simulink model "Trafo_SIMULINK"  (R2022b)
settings: Solver=FixedStepAuto  StartTime=0.0  StopTime=5  FixedStep=0.00001  RelTol=1e-3
values from neighbouring files (symbols this model uses):
  Ct = 1/(Xt*2*pi*f)    (= 9.94718394324e-05)    [Trafo.m]
  k12 = 120/240    (= 0.5)    [Trafo.m]
  k21 = 240/120    (= 2)    [Trafo.m]
  L12 = 0.149*10^-3    (= 0.000149)    [Trafo.m]
  Lm = 1.88    [Trafo.m]
  Lt = Xt/(2*pi*f)    (= 0.101859163579)    [Trafo.m]
  r1 = 0.25    [Trafo.m]
  r2 = 0.134    [Trafo.m]
  Rt = 32    [Trafo.m]
  Umax = 220    [Trafo.m]
  w = 2*pi*50    (= 314.159265359)    [Trafo.m]
settings Model: Creator=Student  LastModifiedBy=petar
settings SolverCC: AlgebraicLoopSolver=TrustRegion
settings DataIOCC: ReturnWorkspaceOutputs=off
settings DebuggingCC: UnconnectedInputMsg=warning  UnconnectedOutputMsg=warning  UnconnectedLineMsg=warning  SFMachineParentedDataDiag=warning  ArithmeticOperatorsInVariantConditions=warning
settings ModelReferenceCC: EnableRefExpFcnMdlSchedulingChecks=on
settings SFSimCC: CustomCodeUndefinedFunction=UseInterfaceOnly

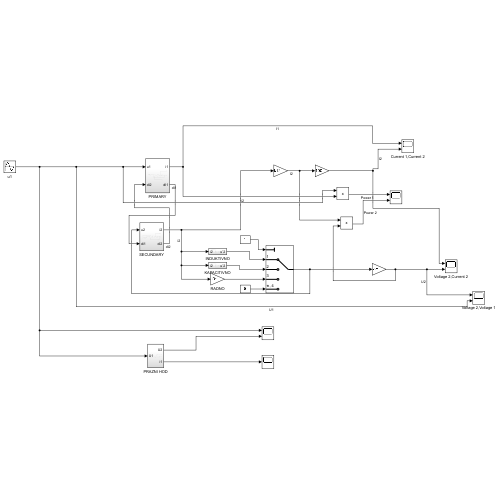
[thumbnail: Simulink's stored preview of the top-level diagram]
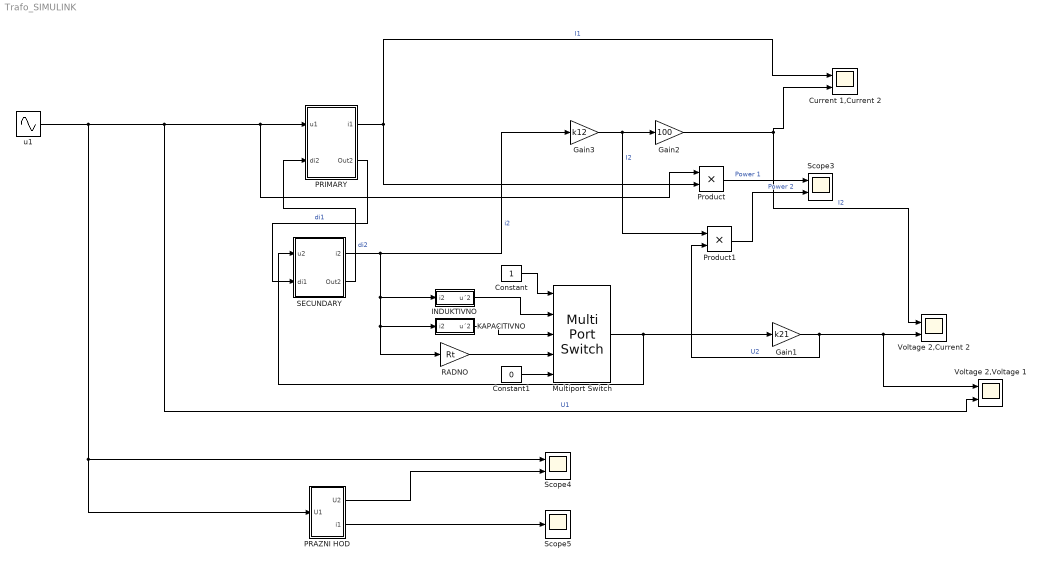
== system Trafo_SIMULINK ==
  Constant : Constant
  Constant1 : Constant  Value=0
  Current 1,Current 2 : Scope  NumInputPorts=2
  Gain1 : Gain  Gain=k21
  Gain2 : Gain  Gain=100
  Gain3 : Gain  Gain=k12
  INDUKTIVNO : Subsystem
  KAPACITIVNO : Subsystem
  Multiport Switch : MultiPortSwitch  Inputs=4  SaturateOnIntegerOverflow=off  InputSameDT=off
  PRAZNI HOD : Subsystem
  PRIMARY : Subsystem
  Product : Product
  Product1 : Product
  RADNO : Gain  Gain=Rt
  SECUNDARY : Subsystem
  Scope3 : Scope  NumInputPorts=2
  Scope4 : Scope  NumInputPorts=2
  Scope5 : Scope
  Voltage 2,Current 2 : Scope  NumInputPorts=2
  Voltage 2,Voltage 1 : Scope  NumInputPorts=2
  u1 : Sin  Amplitude=Umax  Frequency=w  SampleTime=0
  wires:
  u1/1 -> Product/1, PRIMARY/1(u1), Voltage 2,Voltage 1/2, PRAZNI HOD/1(U1), Scope4/1  "U1"
  Gain1/1 -> Product1/2, Voltage 2,Current 2/2, Voltage 2,Voltage 1/1  "U2"
  Gain3/1 -> Product1/1, Gain2/1  "I2"
  PRIMARY/1(i1) -> Current 1,Current 2/1, Product/2  "I1"
  SECUNDARY/1(i2) -> RADNO/1, KAPACITIVNO/1(i2), INDUKTIVNO/1(i2), Gain3/1  "i2"
  PRIMARY/2(Out2) -> SECUNDARY/2(di1)  "di1"
  SECUNDARY/2(Out2) -> PRIMARY/2(di2)  "di2"
  KAPACITIVNO/1(u´2) -> Multiport Switch/3
  INDUKTIVNO/1(u´2) -> Multiport Switch/2
  Multiport Switch/1 -> SECUNDARY/1(u2), Gain1/1
  RADNO/1 -> Multiport Switch/4
  Constant/1 -> Multiport Switch/1
  Gain2/1 -> Current 1,Current 2/2, Voltage 2,Current 2/1  "I2"
  Constant1/1 -> Multiport Switch/5
  Product/1 -> Scope3/1  "Power 1"
  Product1/1 -> Scope3/2  "Power 2"
  PRAZNI HOD/1(U2) -> Scope4/2
  PRAZNI HOD/2(i1) -> Scope5/1

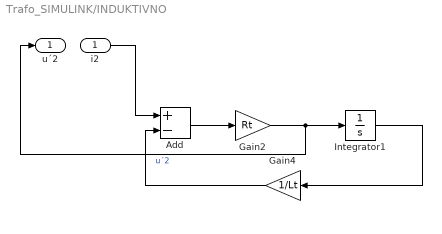
== system Trafo_SIMULINK/INDUKTIVNO ==
  i2 : Inport
  Add : Sum  Inputs=+-
  Gain2 : Gain  Gain=Rt
  Gain4 : Gain  Gain=1/Lt
  Integrator1 : Integrator
  u´2 : Outport  VectorParamsAs1DForOutWhenUnconnected=off
  wires:
  Gain4/1 -> Add/2
  Integrator1/1 -> Gain4/1
  Gain2/1 -> u´2/1, Integrator1/1  "u´2"
  Add/1 -> Gain2/1
  i2/1 -> Add/1

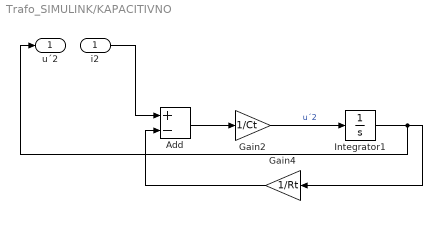
== system Trafo_SIMULINK/KAPACITIVNO ==
  i2 : Inport
  Add : Sum  Inputs=+-
  Gain2 : Gain  Gain=1/Ct
  Gain4 : Gain  Gain=1/Rt
  Integrator1 : Integrator
  u´2 : Outport  VectorParamsAs1DForOutWhenUnconnected=off
  wires:
  Gain4/1 -> Add/2
  Integrator1/1 -> u´2/1, Gain4/1
  Gain2/1 -> Integrator1/1  "u´2"
  Add/1 -> Gain2/1
  i2/1 -> Add/1

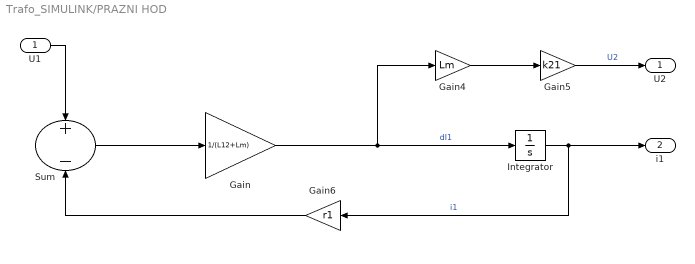
== system Trafo_SIMULINK/PRAZNI HOD ==
  U1 : Inport
  Gain : Gain  Gain=1/(L12+Lm)
  Gain4 : Gain  Gain=Lm
  Gain5 : Gain  Gain=k21
  Gain6 : Gain  Gain=r1
  Integrator : Integrator
  Sum : Sum  Inputs=+-
  U2 : Outport  VectorParamsAs1DForOutWhenUnconnected=off
  i1 : Outport  Port=2  VectorParamsAs1DForOutWhenUnconnected=off
  wires:
  Gain4/1 -> Gain5/1
  Sum/1 -> Gain/1
  Gain6/1 -> Sum/2
  Gain5/1 -> U2/1  "U2"
  Gain/1 -> Gain4/1, Integrator/1  "dI1"
  Integrator/1 -> i1/1, Gain6/1  "i1"
  U1/1 -> Sum/1

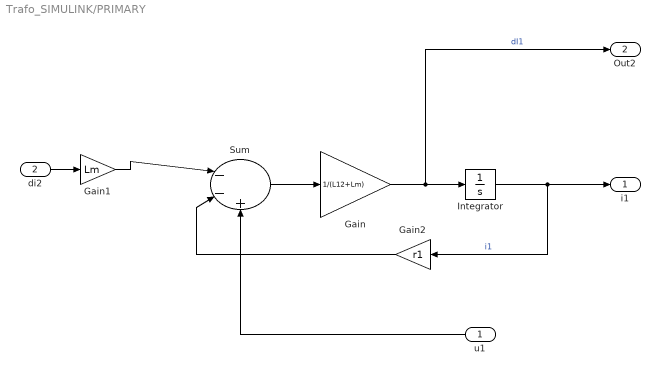
== system Trafo_SIMULINK/PRIMARY ==
  u1 : Inport
  di2 : Inport  Port=2
  Gain : Gain  Gain=1/(L12+Lm)
  Gain1 : Gain  Gain=Lm
  Gain2 : Gain  Gain=r1
  Integrator : Integrator
  Sum : Sum  Inputs=|--+
  i1 : Outport  VectorParamsAs1DForOutWhenUnconnected=off
  Out2 : Outport  Port=2  VectorParamsAs1DForOutWhenUnconnected=off
  wires:
  Gain2/1 -> Sum/2
  Sum/1 -> Gain/1
  Gain/1 -> Out2/1, Integrator/1  "dI1"
  Integrator/1 -> i1/1, Gain2/1  "i1"
  di2/1 -> Gain1/1
  u1/1 -> Sum/3
  Gain1/1 -> Sum/1

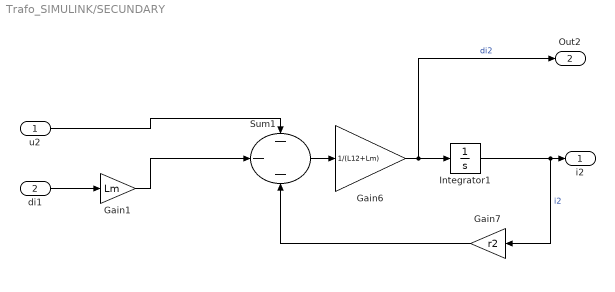
== system Trafo_SIMULINK/SECUNDARY ==
  u2 : Inport
  di1 : Inport  Port=2
  Gain1 : Gain  Gain=Lm
  Gain6 : Gain  Gain=1/(L12+Lm)
  Gain7 : Gain  Gain=r2
  Integrator1 : Integrator
  Sum1 : Sum  Inputs=---
  i2 : Outport  VectorParamsAs1DForOutWhenUnconnected=off
  Out2 : Outport  Port=2  VectorParamsAs1DForOutWhenUnconnected=off
  wires:
  Gain7/1 -> Sum1/3
  Integrator1/1 -> Gain7/1, i2/1  "i2"
  di1/1 -> Gain1/1
  Gain6/1 -> Out2/1, Integrator1/1  "di2"
  Sum1/1 -> Gain6/1
  u2/1 -> Sum1/1
  Gain1/1 -> Sum1/2
